simulink model "gm_hybrid_lht"  (R2019b)
settings: Solver=FixedStepDiscrete  StartTime=0.0  StopTime=inf  FixedStep=1/120e6  RelTol=1e-3
undefined symbols (not defined in the file or in its folder): bt, height, nTheta, width
libraries: hdlsllib x352, simulink x286, hdlmdlgenlib x7, dspsrcs4 x1
(part 2 of 12)

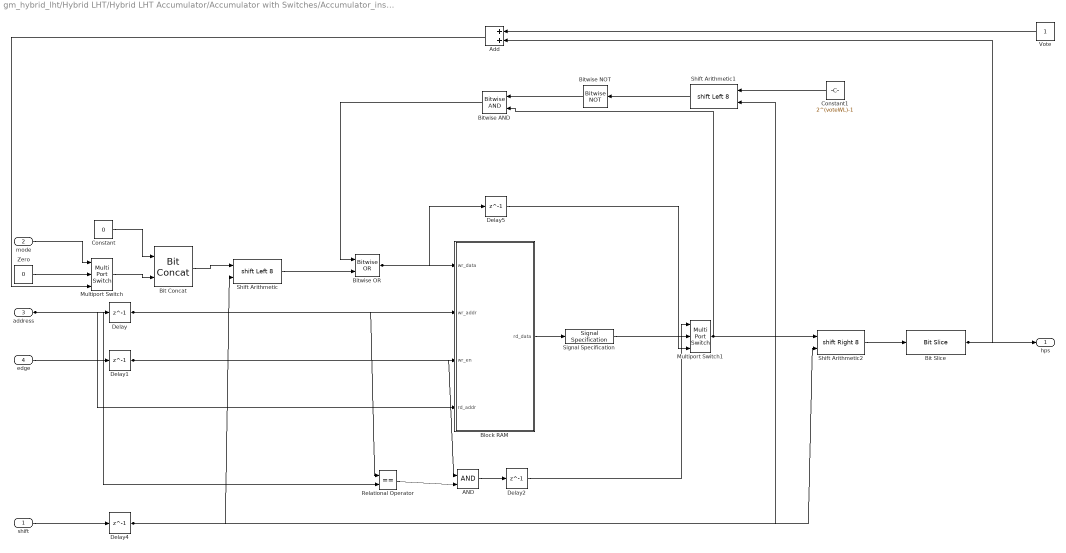
== system gm_hybrid_lht/Hybrid LHT/Hybrid LHT Accumulator/Accumulator with Switches/Accumulator_instance1 ==
  shift : Inport  OutDataTypeStr=fixdt(0, 6, 0)  PortDimensions=1  SampleTime=8.33333333333333e-09
  mode : Inport  Port=2  OutDataTypeStr=boolean  PortDimensions=1  SampleTime=8.33333333333333e-09
  address : Inport  Port=3  OutDataTypeStr=fixdt(0, 11, 0)  PortDimensions=1  SampleTime=8.33333333333333e-09
  edge : Inport  Port=4  OutDataTypeStr=boolean  PortDimensions=1  SampleTime=8.33333333333333e-09
  AND : Logic  IconShape=distinctive  AllPortsSameDT=off  OutDataTypeStr=boolean
  Add : Sum  OutDataTypeStr=fixdt(0, ceil(log2(maxRho*2)), 0)
  Bit Concat : hdlsllib/Logic and Bit Operations/Bit Concat  numInputs=2
      settings: SourceProductName=Simulink
  Bit Slice : hdlsllib/Logic and Bit Operations/Bit Slice  lidx=voteWL-1  ridx=0
  Bitwise AND : simulink/Logic and Bit Operations/Bitwise Operator  logicop=AND  UseBitMask=off  NumInputPorts=2  BitMask=bin2dec('11011001')  BitMaskRealWorld=Stored Integer
  Bitwise NOT : simulink/Logic and Bit Operations/Bitwise Operator  logicop=NOT  UseBitMask=off  BitMask=bin2dec('11011001')  BitMaskRealWorld=Stored Integer
  Bitwise OR : simulink/Logic and Bit Operations/Bitwise Operator  logicop=OR  UseBitMask=off  NumInputPorts=2  BitMask=bin2dec('11011001')  BitMaskRealWorld=Stored Integer
  Block RAM : Subsystem
  Constant : Constant  Value=0  OutDataTypeStr=fixdt(0, 36-voteWL, 0)  SampleTime=-1
  Constant1 : Constant  Value=2^(voteWL)-1  OutDataTypeStr=fixdt(0, 36, 0)  SampleTime=-1
  Delay{,1..2,4..5} (5 alike) : Delay  DelayLength=1
  Multiport Switch : MultiPortSwitch  DataPortOrder=Zero-based contiguous  Inputs=2  zeroidx=on
  Multiport Switch1 : MultiPortSwitch  DataPortOrder=Zero-based contiguous  Inputs=2  zeroidx=on
  Relational Operator : RelationalOperator  Operator===  OutDataTypeStr=boolean  RndMeth=Simplest
  Shift Arithmetic : ArithShift  BitShiftNumberSource=Input port  BitShiftNumber=8  BitShiftDirection=Left  DiagnosticForOORShift=Error
      settings: InputPortMap=u0,p1
  Shift Arithmetic1 : ArithShift  BitShiftNumberSource=Input port  BitShiftNumber=8  BitShiftDirection=Left  DiagnosticForOORShift=Error
      settings: InputPortMap=u0,p1
  Shift Arithmetic2 : ArithShift  BitShiftNumberSource=Input port  BitShiftNumber=8  BitShiftDirection=Right  DiagnosticForOORShift=Error
      settings: InputPortMap=u0,p1
  Signal Specification : SignalSpecification  OutDataTypeStr=fixdt(0, 36, 0)
  Vote : Constant  OutDataTypeStr=fixdt(0,1,0)  SampleTime=-1
  Zero : Constant  Value=0  OutDataTypeStr=fixdt(0,1,0)  SampleTime=-1
  hps : Outport
  wires:
  Zero/1 -> Multiport Switch/2
  Vote/1 -> Add/1
  Shift Arithmetic1/1 -> Bitwise NOT/1
  Relational Operator/1 -> AND/2
  Delay4/1 -> Shift Arithmetic1/2, Shift Arithmetic/2, Shift Arithmetic2/2
  Delay2/1 -> Multiport Switch1/1
  Delay1/1 -> AND/1, Block RAM/3(wr_en)
  Delay/1 -> Relational Operator/1, Block RAM/2(wr_addr)
  Constant1/1 -> Shift Arithmetic1/1
  Constant/1 -> Bit Concat/1
  Bitwise NOT/1 -> Bitwise AND/1
  Bit Slice/1 -> hps/1, Add/2
  AND/1 -> Delay2/1
  shift/1 -> Delay4/1
  mode/1 -> Multiport Switch/1
  address/1 -> Relational Operator/2, Delay/1, Block RAM/4(rd_addr)
  edge/1 -> Delay1/1
  Delay5/1 -> Multiport Switch1/3
  Shift Arithmetic/1 -> Bitwise OR/2
  Bit Concat/1 -> Shift Arithmetic/1
  Multiport Switch/1 -> Bit Concat/2
  Add/1 -> Multiport Switch/3
  Shift Arithmetic2/1 -> Bit Slice/1
  Bitwise AND/1 -> Bitwise OR/1
  Bitwise OR/1 -> Delay5/1, Block RAM/1(wr_data)
  Signal Specification/1 -> Multiport Switch1/2
  Multiport Switch1/1 -> Bitwise AND/2, Shift Arithmetic2/1
  Block RAM/1(rd_data) -> Signal Specification/1

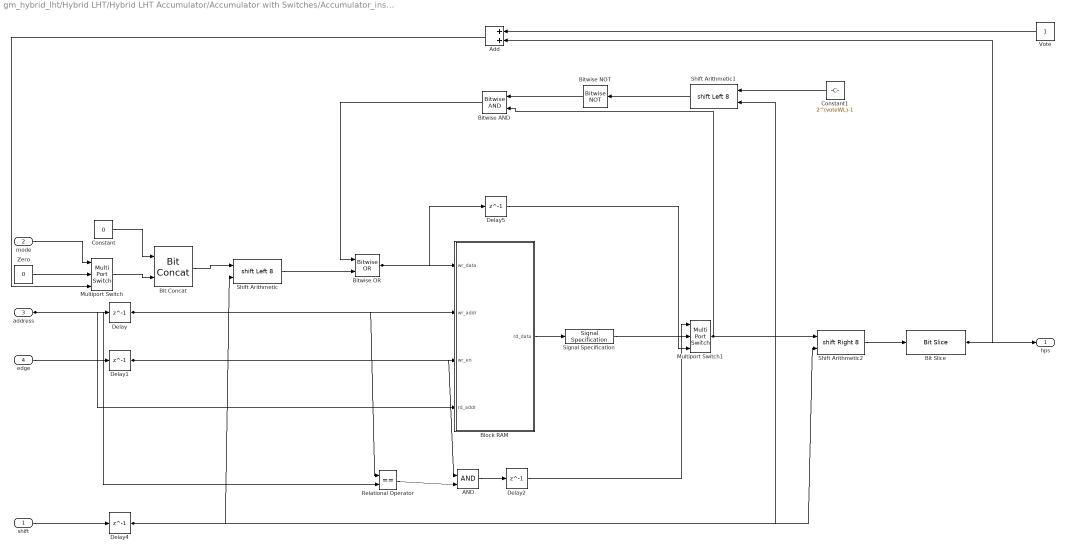
== system gm_hybrid_lht/Hybrid LHT/Hybrid LHT Accumulator/Accumulator with Switches/Accumulator_instance10 ==
  shift : Inport  OutDataTypeStr=fixdt(0, 6, 0)  PortDimensions=1  SampleTime=8.33333333333333e-09
  mode : Inport  Port=2  OutDataTypeStr=boolean  PortDimensions=1  SampleTime=8.33333333333333e-09
  address : Inport  Port=3  OutDataTypeStr=fixdt(0, 11, 0)  PortDimensions=1  SampleTime=8.33333333333333e-09
  edge : Inport  Port=4  OutDataTypeStr=boolean  PortDimensions=1  SampleTime=8.33333333333333e-09
  AND : Logic  IconShape=distinctive  AllPortsSameDT=off  OutDataTypeStr=boolean
  Add : Sum  OutDataTypeStr=fixdt(0, ceil(log2(maxRho*2)), 0)
  Bit Concat : hdlsllib/Logic and Bit Operations/Bit Concat  numInputs=2
      settings: SourceProductName=Simulink
  Bit Slice : hdlsllib/Logic and Bit Operations/Bit Slice  lidx=voteWL-1  ridx=0
  Bitwise AND : simulink/Logic and Bit Operations/Bitwise Operator  logicop=AND  UseBitMask=off  NumInputPorts=2  BitMask=bin2dec('11011001')  BitMaskRealWorld=Stored Integer
  Bitwise NOT : simulink/Logic and Bit Operations/Bitwise Operator  logicop=NOT  UseBitMask=off  BitMask=bin2dec('11011001')  BitMaskRealWorld=Stored Integer
  Bitwise OR : simulink/Logic and Bit Operations/Bitwise Operator  logicop=OR  UseBitMask=off  NumInputPorts=2  BitMask=bin2dec('11011001')  BitMaskRealWorld=Stored Integer
  Block RAM : Subsystem
  Constant : Constant  Value=0  OutDataTypeStr=fixdt(0, 36-voteWL, 0)  SampleTime=-1
  Constant1 : Constant  Value=2^(voteWL)-1  OutDataTypeStr=fixdt(0, 36, 0)  SampleTime=-1
  Delay{,1..2,4..5} (5 alike) : Delay  DelayLength=1
  Multiport Switch : MultiPortSwitch  DataPortOrder=Zero-based contiguous  Inputs=2  zeroidx=on
  Multiport Switch1 : MultiPortSwitch  DataPortOrder=Zero-based contiguous  Inputs=2  zeroidx=on
  Relational Operator : RelationalOperator  Operator===  OutDataTypeStr=boolean  RndMeth=Simplest
  Shift Arithmetic : ArithShift  BitShiftNumberSource=Input port  BitShiftNumber=8  BitShiftDirection=Left  DiagnosticForOORShift=Error
      settings: InputPortMap=u0,p1
  Shift Arithmetic1 : ArithShift  BitShiftNumberSource=Input port  BitShiftNumber=8  BitShiftDirection=Left  DiagnosticForOORShift=Error
      settings: InputPortMap=u0,p1
  Shift Arithmetic2 : ArithShift  BitShiftNumberSource=Input port  BitShiftNumber=8  BitShiftDirection=Right  DiagnosticForOORShift=Error
      settings: InputPortMap=u0,p1
  Signal Specification : SignalSpecification  OutDataTypeStr=fixdt(0, 36, 0)
  Vote : Constant  OutDataTypeStr=fixdt(0,1,0)  SampleTime=-1
  Zero : Constant  Value=0  OutDataTypeStr=fixdt(0,1,0)  SampleTime=-1
  hps : Outport
  wires:
  Block RAM/1(rd_data) -> Signal Specification/1
  Multiport Switch1/1 -> Shift Arithmetic2/1, Bitwise AND/2
  Signal Specification/1 -> Multiport Switch1/2
  Bitwise OR/1 -> Block RAM/1(wr_data), Delay5/1
  Bitwise AND/1 -> Bitwise OR/1
  Shift Arithmetic2/1 -> Bit Slice/1
  Add/1 -> Multiport Switch/3
  Multiport Switch/1 -> Bit Concat/2
  Bit Concat/1 -> Shift Arithmetic/1
  Shift Arithmetic/1 -> Bitwise OR/2
  Delay5/1 -> Multiport Switch1/3
  edge/1 -> Delay1/1
  address/1 -> Block RAM/4(rd_addr), Delay/1, Relational Operator/2
  mode/1 -> Multiport Switch/1
  shift/1 -> Delay4/1
  AND/1 -> Delay2/1
  Bit Slice/1 -> Add/2, hps/1
  Bitwise NOT/1 -> Bitwise AND/1
  Constant/1 -> Bit Concat/1
  Constant1/1 -> Shift Arithmetic1/1
  Delay/1 -> Block RAM/2(wr_addr), Relational Operator/1
  Delay1/1 -> Block RAM/3(wr_en), AND/1
  Delay2/1 -> Multiport Switch1/1
  Delay4/1 -> Shift Arithmetic2/2, Shift Arithmetic/2, Shift Arithmetic1/2
  Relational Operator/1 -> AND/2
  Shift Arithmetic1/1 -> Bitwise NOT/1
  Vote/1 -> Add/1
  Zero/1 -> Multiport Switch/2

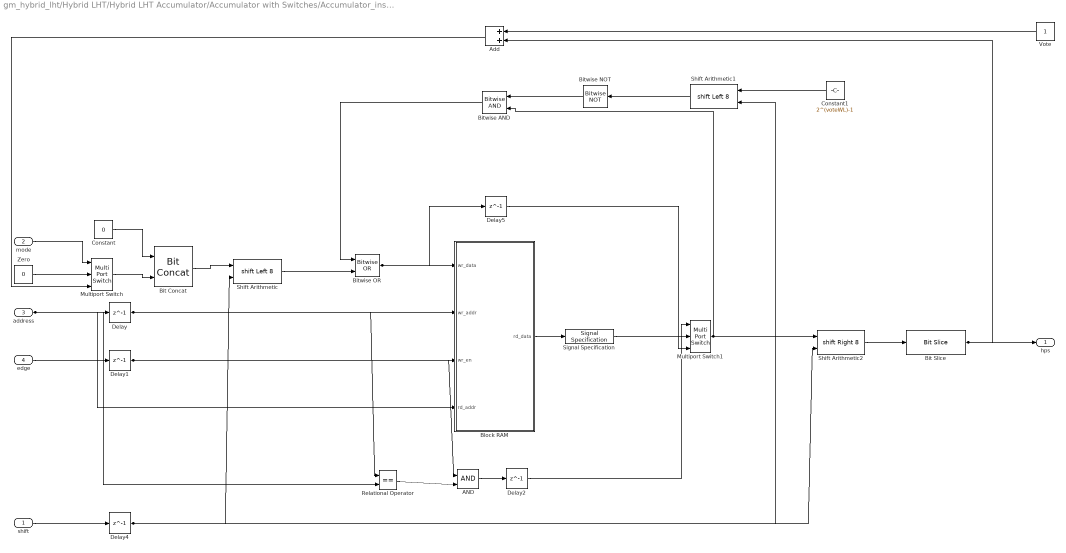
== system gm_hybrid_lht/Hybrid LHT/Hybrid LHT Accumulator/Accumulator with Switches/Accumulator_instance11 ==
  shift : Inport  OutDataTypeStr=fixdt(0, 6, 0)  PortDimensions=1  SampleTime=8.33333333333333e-09
  mode : Inport  Port=2  OutDataTypeStr=boolean  PortDimensions=1  SampleTime=8.33333333333333e-09
  address : Inport  Port=3  OutDataTypeStr=fixdt(0, 11, 0)  PortDimensions=1  SampleTime=8.33333333333333e-09
  edge : Inport  Port=4  OutDataTypeStr=boolean  PortDimensions=1  SampleTime=8.33333333333333e-09
  AND : Logic  IconShape=distinctive  AllPortsSameDT=off  OutDataTypeStr=boolean
  Add : Sum  OutDataTypeStr=fixdt(0, ceil(log2(maxRho*2)), 0)
  Bit Concat : hdlsllib/Logic and Bit Operations/Bit Concat  numInputs=2
      settings: SourceProductName=Simulink
  Bit Slice : hdlsllib/Logic and Bit Operations/Bit Slice  lidx=voteWL-1  ridx=0
  Bitwise AND : simulink/Logic and Bit Operations/Bitwise Operator  logicop=AND  UseBitMask=off  NumInputPorts=2  BitMask=bin2dec('11011001')  BitMaskRealWorld=Stored Integer
  Bitwise NOT : simulink/Logic and Bit Operations/Bitwise Operator  logicop=NOT  UseBitMask=off  BitMask=bin2dec('11011001')  BitMaskRealWorld=Stored Integer
  Bitwise OR : simulink/Logic and Bit Operations/Bitwise Operator  logicop=OR  UseBitMask=off  NumInputPorts=2  BitMask=bin2dec('11011001')  BitMaskRealWorld=Stored Integer
  Block RAM : Subsystem
  Constant : Constant  Value=0  OutDataTypeStr=fixdt(0, 36-voteWL, 0)  SampleTime=-1
  Constant1 : Constant  Value=2^(voteWL)-1  OutDataTypeStr=fixdt(0, 36, 0)  SampleTime=-1
  Delay{,1..2,4..5} (5 alike) : Delay  DelayLength=1
  Multiport Switch : MultiPortSwitch  DataPortOrder=Zero-based contiguous  Inputs=2  zeroidx=on
  Multiport Switch1 : MultiPortSwitch  DataPortOrder=Zero-based contiguous  Inputs=2  zeroidx=on
  Relational Operator : RelationalOperator  Operator===  OutDataTypeStr=boolean  RndMeth=Simplest
  Shift Arithmetic : ArithShift  BitShiftNumberSource=Input port  BitShiftNumber=8  BitShiftDirection=Left  DiagnosticForOORShift=Error
      settings: InputPortMap=u0,p1
  Shift Arithmetic1 : ArithShift  BitShiftNumberSource=Input port  BitShiftNumber=8  BitShiftDirection=Left  DiagnosticForOORShift=Error
      settings: InputPortMap=u0,p1
  Shift Arithmetic2 : ArithShift  BitShiftNumberSource=Input port  BitShiftNumber=8  BitShiftDirection=Right  DiagnosticForOORShift=Error
      settings: InputPortMap=u0,p1
  Signal Specification : SignalSpecification  OutDataTypeStr=fixdt(0, 36, 0)
  Vote : Constant  OutDataTypeStr=fixdt(0,1,0)  SampleTime=-1
  Zero : Constant  Value=0  OutDataTypeStr=fixdt(0,1,0)  SampleTime=-1
  hps : Outport
  wires:
  Block RAM/1(rd_data) -> Signal Specification/1
  Multiport Switch1/1 -> Shift Arithmetic2/1, Bitwise AND/2
  Signal Specification/1 -> Multiport Switch1/2
  Bitwise OR/1 -> Block RAM/1(wr_data), Delay5/1
  Bitwise AND/1 -> Bitwise OR/1
  Shift Arithmetic2/1 -> Bit Slice/1
  Add/1 -> Multiport Switch/3
  Multiport Switch/1 -> Bit Concat/2
  Bit Concat/1 -> Shift Arithmetic/1
  Shift Arithmetic/1 -> Bitwise OR/2
  Delay5/1 -> Multiport Switch1/3
  edge/1 -> Delay1/1
  address/1 -> Block RAM/4(rd_addr), Delay/1, Relational Operator/2
  mode/1 -> Multiport Switch/1
  shift/1 -> Delay4/1
  AND/1 -> Delay2/1
  Bit Slice/1 -> Add/2, hps/1
  Bitwise NOT/1 -> Bitwise AND/1
  Constant/1 -> Bit Concat/1
  Constant1/1 -> Shift Arithmetic1/1
  Delay/1 -> Block RAM/2(wr_addr), Relational Operator/1
  Delay1/1 -> Block RAM/3(wr_en), AND/1
  Delay2/1 -> Multiport Switch1/1
  Delay4/1 -> Shift Arithmetic2/2, Shift Arithmetic/2, Shift Arithmetic1/2
  Relational Operator/1 -> AND/2
  Shift Arithmetic1/1 -> Bitwise NOT/1
  Vote/1 -> Add/1
  Zero/1 -> Multiport Switch/2

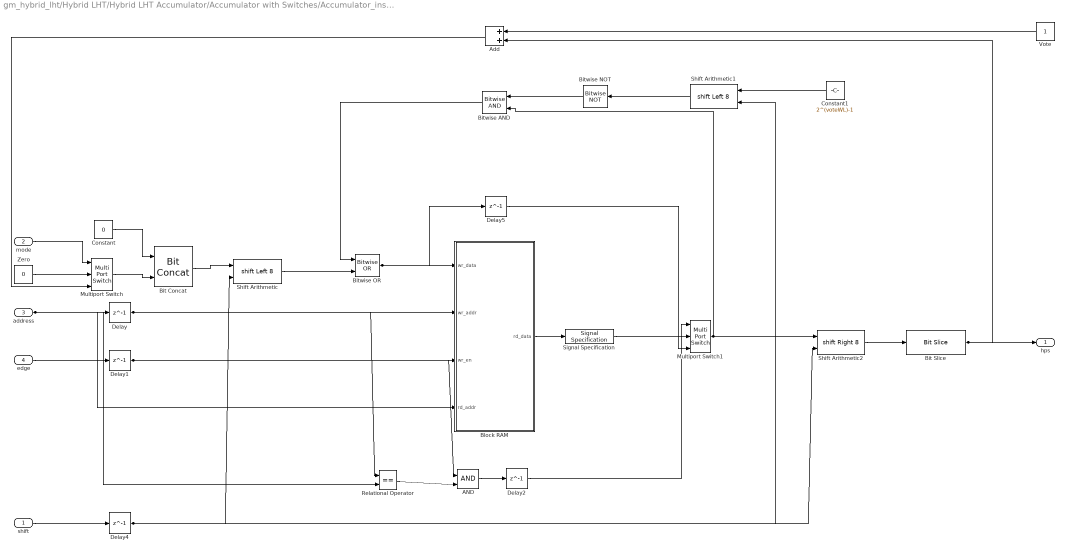
== system gm_hybrid_lht/Hybrid LHT/Hybrid LHT Accumulator/Accumulator with Switches/Accumulator_instance12 ==
  shift : Inport  OutDataTypeStr=fixdt(0, 6, 0)  PortDimensions=1  SampleTime=8.33333333333333e-09
  mode : Inport  Port=2  OutDataTypeStr=boolean  PortDimensions=1  SampleTime=8.33333333333333e-09
  address : Inport  Port=3  OutDataTypeStr=fixdt(0, 11, 0)  PortDimensions=1  SampleTime=8.33333333333333e-09
  edge : Inport  Port=4  OutDataTypeStr=boolean  PortDimensions=1  SampleTime=8.33333333333333e-09
  AND : Logic  IconShape=distinctive  AllPortsSameDT=off  OutDataTypeStr=boolean
  Add : Sum  OutDataTypeStr=fixdt(0, ceil(log2(maxRho*2)), 0)
  Bit Concat : hdlsllib/Logic and Bit Operations/Bit Concat  numInputs=2
      settings: SourceProductName=Simulink
  Bit Slice : hdlsllib/Logic and Bit Operations/Bit Slice  lidx=voteWL-1  ridx=0
  Bitwise AND : simulink/Logic and Bit Operations/Bitwise Operator  logicop=AND  UseBitMask=off  NumInputPorts=2  BitMask=bin2dec('11011001')  BitMaskRealWorld=Stored Integer
  Bitwise NOT : simulink/Logic and Bit Operations/Bitwise Operator  logicop=NOT  UseBitMask=off  BitMask=bin2dec('11011001')  BitMaskRealWorld=Stored Integer
  Bitwise OR : simulink/Logic and Bit Operations/Bitwise Operator  logicop=OR  UseBitMask=off  NumInputPorts=2  BitMask=bin2dec('11011001')  BitMaskRealWorld=Stored Integer
  Block RAM : Subsystem
  Constant : Constant  Value=0  OutDataTypeStr=fixdt(0, 36-voteWL, 0)  SampleTime=-1
  Constant1 : Constant  Value=2^(voteWL)-1  OutDataTypeStr=fixdt(0, 36, 0)  SampleTime=-1
  Delay{,1..2,4..5} (5 alike) : Delay  DelayLength=1
  Multiport Switch : MultiPortSwitch  DataPortOrder=Zero-based contiguous  Inputs=2  zeroidx=on
  Multiport Switch1 : MultiPortSwitch  DataPortOrder=Zero-based contiguous  Inputs=2  zeroidx=on
  Relational Operator : RelationalOperator  Operator===  OutDataTypeStr=boolean  RndMeth=Simplest
  Shift Arithmetic : ArithShift  BitShiftNumberSource=Input port  BitShiftNumber=8  BitShiftDirection=Left  DiagnosticForOORShift=Error
      settings: InputPortMap=u0,p1
  Shift Arithmetic1 : ArithShift  BitShiftNumberSource=Input port  BitShiftNumber=8  BitShiftDirection=Left  DiagnosticForOORShift=Error
      settings: InputPortMap=u0,p1
  Shift Arithmetic2 : ArithShift  BitShiftNumberSource=Input port  BitShiftNumber=8  BitShiftDirection=Right  DiagnosticForOORShift=Error
      settings: InputPortMap=u0,p1
  Signal Specification : SignalSpecification  OutDataTypeStr=fixdt(0, 36, 0)
  Vote : Constant  OutDataTypeStr=fixdt(0,1,0)  SampleTime=-1
  Zero : Constant  Value=0  OutDataTypeStr=fixdt(0,1,0)  SampleTime=-1
  hps : Outport
  wires:
  Block RAM/1(rd_data) -> Signal Specification/1
  Multiport Switch1/1 -> Shift Arithmetic2/1, Bitwise AND/2
  Signal Specification/1 -> Multiport Switch1/2
  Bitwise OR/1 -> Block RAM/1(wr_data), Delay5/1
  Bitwise AND/1 -> Bitwise OR/1
  Shift Arithmetic2/1 -> Bit Slice/1
  Add/1 -> Multiport Switch/3
  Multiport Switch/1 -> Bit Concat/2
  Bit Concat/1 -> Shift Arithmetic/1
  Shift Arithmetic/1 -> Bitwise OR/2
  Delay5/1 -> Multiport Switch1/3
  edge/1 -> Delay1/1
  address/1 -> Block RAM/4(rd_addr), Delay/1, Relational Operator/2
  mode/1 -> Multiport Switch/1
  shift/1 -> Delay4/1
  AND/1 -> Delay2/1
  Bit Slice/1 -> Add/2, hps/1
  Bitwise NOT/1 -> Bitwise AND/1
  Constant/1 -> Bit Concat/1
  Constant1/1 -> Shift Arithmetic1/1
  Delay/1 -> Block RAM/2(wr_addr), Relational Operator/1
  Delay1/1 -> Block RAM/3(wr_en), AND/1
  Delay2/1 -> Multiport Switch1/1
  Delay4/1 -> Shift Arithmetic2/2, Shift Arithmetic/2, Shift Arithmetic1/2
  Relational Operator/1 -> AND/2
  Shift Arithmetic1/1 -> Bitwise NOT/1
  Vote/1 -> Add/1
  Zero/1 -> Multiport Switch/2

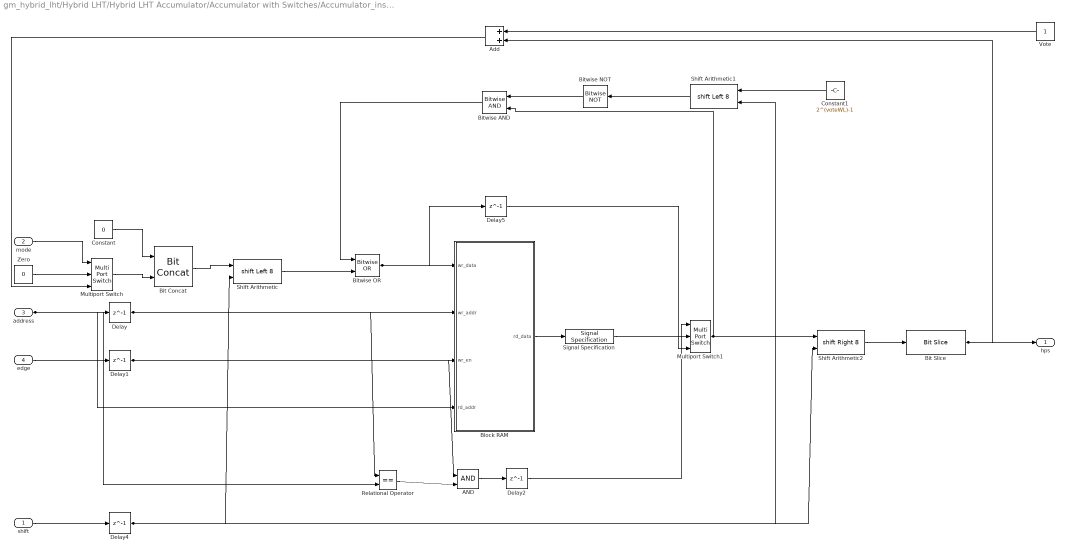
== system gm_hybrid_lht/Hybrid LHT/Hybrid LHT Accumulator/Accumulator with Switches/Accumulator_instance13 ==
  shift : Inport  OutDataTypeStr=fixdt(0, 6, 0)  PortDimensions=1  SampleTime=8.33333333333333e-09
  mode : Inport  Port=2  OutDataTypeStr=boolean  PortDimensions=1  SampleTime=8.33333333333333e-09
  address : Inport  Port=3  OutDataTypeStr=fixdt(0, 11, 0)  PortDimensions=1  SampleTime=8.33333333333333e-09
  edge : Inport  Port=4  OutDataTypeStr=boolean  PortDimensions=1  SampleTime=8.33333333333333e-09
  AND : Logic  IconShape=distinctive  AllPortsSameDT=off  OutDataTypeStr=boolean
  Add : Sum  OutDataTypeStr=fixdt(0, ceil(log2(maxRho*2)), 0)
  Bit Concat : hdlsllib/Logic and Bit Operations/Bit Concat  numInputs=2
      settings: SourceProductName=Simulink
  Bit Slice : hdlsllib/Logic and Bit Operations/Bit Slice  lidx=voteWL-1  ridx=0
  Bitwise AND : simulink/Logic and Bit Operations/Bitwise Operator  logicop=AND  UseBitMask=off  NumInputPorts=2  BitMask=bin2dec('11011001')  BitMaskRealWorld=Stored Integer
  Bitwise NOT : simulink/Logic and Bit Operations/Bitwise Operator  logicop=NOT  UseBitMask=off  BitMask=bin2dec('11011001')  BitMaskRealWorld=Stored Integer
  Bitwise OR : simulink/Logic and Bit Operations/Bitwise Operator  logicop=OR  UseBitMask=off  NumInputPorts=2  BitMask=bin2dec('11011001')  BitMaskRealWorld=Stored Integer
  Block RAM : Subsystem
  Constant : Constant  Value=0  OutDataTypeStr=fixdt(0, 36-voteWL, 0)  SampleTime=-1
  Constant1 : Constant  Value=2^(voteWL)-1  OutDataTypeStr=fixdt(0, 36, 0)  SampleTime=-1
  Delay{,1..2,4..5} (5 alike) : Delay  DelayLength=1
  Multiport Switch : MultiPortSwitch  DataPortOrder=Zero-based contiguous  Inputs=2  zeroidx=on
  Multiport Switch1 : MultiPortSwitch  DataPortOrder=Zero-based contiguous  Inputs=2  zeroidx=on
  Relational Operator : RelationalOperator  Operator===  OutDataTypeStr=boolean  RndMeth=Simplest
  Shift Arithmetic : ArithShift  BitShiftNumberSource=Input port  BitShiftNumber=8  BitShiftDirection=Left  DiagnosticForOORShift=Error
      settings: InputPortMap=u0,p1
  Shift Arithmetic1 : ArithShift  BitShiftNumberSource=Input port  BitShiftNumber=8  BitShiftDirection=Left  DiagnosticForOORShift=Error
      settings: InputPortMap=u0,p1
  Shift Arithmetic2 : ArithShift  BitShiftNumberSource=Input port  BitShiftNumber=8  BitShiftDirection=Right  DiagnosticForOORShift=Error
      settings: InputPortMap=u0,p1
  Signal Specification : SignalSpecification  OutDataTypeStr=fixdt(0, 36, 0)
  Vote : Constant  OutDataTypeStr=fixdt(0,1,0)  SampleTime=-1
  Zero : Constant  Value=0  OutDataTypeStr=fixdt(0,1,0)  SampleTime=-1
  hps : Outport
  wires:
  Block RAM/1(rd_data) -> Signal Specification/1
  Multiport Switch1/1 -> Shift Arithmetic2/1, Bitwise AND/2
  Signal Specification/1 -> Multiport Switch1/2
  Bitwise OR/1 -> Block RAM/1(wr_data), Delay5/1
  Bitwise AND/1 -> Bitwise OR/1
  Shift Arithmetic2/1 -> Bit Slice/1
  Add/1 -> Multiport Switch/3
  Multiport Switch/1 -> Bit Concat/2
  Bit Concat/1 -> Shift Arithmetic/1
  Shift Arithmetic/1 -> Bitwise OR/2
  Delay5/1 -> Multiport Switch1/3
  edge/1 -> Delay1/1
  address/1 -> Block RAM/4(rd_addr), Delay/1, Relational Operator/2
  mode/1 -> Multiport Switch/1
  shift/1 -> Delay4/1
  AND/1 -> Delay2/1
  Bit Slice/1 -> Add/2, hps/1
  Bitwise NOT/1 -> Bitwise AND/1
  Constant/1 -> Bit Concat/1
  Constant1/1 -> Shift Arithmetic1/1
  Delay/1 -> Block RAM/2(wr_addr), Relational Operator/1
  Delay1/1 -> Block RAM/3(wr_en), AND/1
  Delay2/1 -> Multiport Switch1/1
  Delay4/1 -> Shift Arithmetic2/2, Shift Arithmetic/2, Shift Arithmetic1/2
  Relational Operator/1 -> AND/2
  Shift Arithmetic1/1 -> Bitwise NOT/1
  Vote/1 -> Add/1
  Zero/1 -> Multiport Switch/2

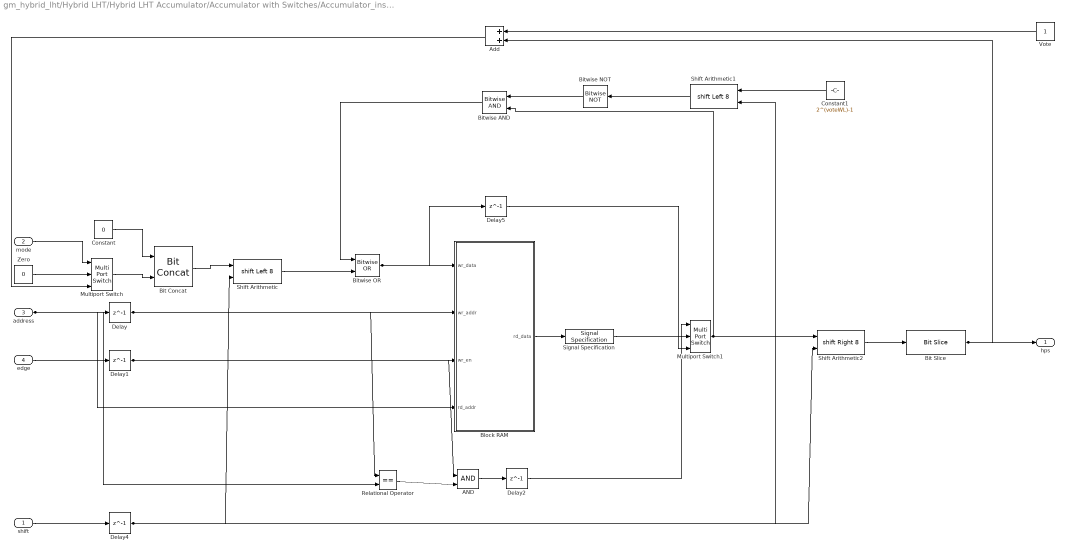
== system gm_hybrid_lht/Hybrid LHT/Hybrid LHT Accumulator/Accumulator with Switches/Accumulator_instance14 ==
  shift : Inport  OutDataTypeStr=fixdt(0, 6, 0)  PortDimensions=1  SampleTime=8.33333333333333e-09
  mode : Inport  Port=2  OutDataTypeStr=boolean  PortDimensions=1  SampleTime=8.33333333333333e-09
  address : Inport  Port=3  OutDataTypeStr=fixdt(0, 11, 0)  PortDimensions=1  SampleTime=8.33333333333333e-09
  edge : Inport  Port=4  OutDataTypeStr=boolean  PortDimensions=1  SampleTime=8.33333333333333e-09
  AND : Logic  IconShape=distinctive  AllPortsSameDT=off  OutDataTypeStr=boolean
  Add : Sum  OutDataTypeStr=fixdt(0, ceil(log2(maxRho*2)), 0)
  Bit Concat : hdlsllib/Logic and Bit Operations/Bit Concat  numInputs=2
      settings: SourceProductName=Simulink
  Bit Slice : hdlsllib/Logic and Bit Operations/Bit Slice  lidx=voteWL-1  ridx=0
  Bitwise AND : simulink/Logic and Bit Operations/Bitwise Operator  logicop=AND  UseBitMask=off  NumInputPorts=2  BitMask=bin2dec('11011001')  BitMaskRealWorld=Stored Integer
  Bitwise NOT : simulink/Logic and Bit Operations/Bitwise Operator  logicop=NOT  UseBitMask=off  BitMask=bin2dec('11011001')  BitMaskRealWorld=Stored Integer
  Bitwise OR : simulink/Logic and Bit Operations/Bitwise Operator  logicop=OR  UseBitMask=off  NumInputPorts=2  BitMask=bin2dec('11011001')  BitMaskRealWorld=Stored Integer
  Block RAM : Subsystem
  Constant : Constant  Value=0  OutDataTypeStr=fixdt(0, 36-voteWL, 0)  SampleTime=-1
  Constant1 : Constant  Value=2^(voteWL)-1  OutDataTypeStr=fixdt(0, 36, 0)  SampleTime=-1
  Delay{,1..2,4..5} (5 alike) : Delay  DelayLength=1
  Multiport Switch : MultiPortSwitch  DataPortOrder=Zero-based contiguous  Inputs=2  zeroidx=on
  Multiport Switch1 : MultiPortSwitch  DataPortOrder=Zero-based contiguous  Inputs=2  zeroidx=on
  Relational Operator : RelationalOperator  Operator===  OutDataTypeStr=boolean  RndMeth=Simplest
  Shift Arithmetic : ArithShift  BitShiftNumberSource=Input port  BitShiftNumber=8  BitShiftDirection=Left  DiagnosticForOORShift=Error
      settings: InputPortMap=u0,p1
  Shift Arithmetic1 : ArithShift  BitShiftNumberSource=Input port  BitShiftNumber=8  BitShiftDirection=Left  DiagnosticForOORShift=Error
      settings: InputPortMap=u0,p1
  Shift Arithmetic2 : ArithShift  BitShiftNumberSource=Input port  BitShiftNumber=8  BitShiftDirection=Right  DiagnosticForOORShift=Error
      settings: InputPortMap=u0,p1
  Signal Specification : SignalSpecification  OutDataTypeStr=fixdt(0, 36, 0)
  Vote : Constant  OutDataTypeStr=fixdt(0,1,0)  SampleTime=-1
  Zero : Constant  Value=0  OutDataTypeStr=fixdt(0,1,0)  SampleTime=-1
  hps : Outport
  wires:
  Block RAM/1(rd_data) -> Signal Specification/1
  Multiport Switch1/1 -> Shift Arithmetic2/1, Bitwise AND/2
  Signal Specification/1 -> Multiport Switch1/2
  Bitwise OR/1 -> Block RAM/1(wr_data), Delay5/1
  Bitwise AND/1 -> Bitwise OR/1
  Shift Arithmetic2/1 -> Bit Slice/1
  Add/1 -> Multiport Switch/3
  Multiport Switch/1 -> Bit Concat/2
  Bit Concat/1 -> Shift Arithmetic/1
  Shift Arithmetic/1 -> Bitwise OR/2
  Delay5/1 -> Multiport Switch1/3
  edge/1 -> Delay1/1
  address/1 -> Block RAM/4(rd_addr), Delay/1, Relational Operator/2
  mode/1 -> Multiport Switch/1
  shift/1 -> Delay4/1
  AND/1 -> Delay2/1
  Bit Slice/1 -> Add/2, hps/1
  Bitwise NOT/1 -> Bitwise AND/1
  Constant/1 -> Bit Concat/1
  Constant1/1 -> Shift Arithmetic1/1
  Delay/1 -> Block RAM/2(wr_addr), Relational Operator/1
  Delay1/1 -> Block RAM/3(wr_en), AND/1
  Delay2/1 -> Multiport Switch1/1
  Delay4/1 -> Shift Arithmetic2/2, Shift Arithmetic/2, Shift Arithmetic1/2
  Relational Operator/1 -> AND/2
  Shift Arithmetic1/1 -> Bitwise NOT/1
  Vote/1 -> Add/1
  Zero/1 -> Multiport Switch/2

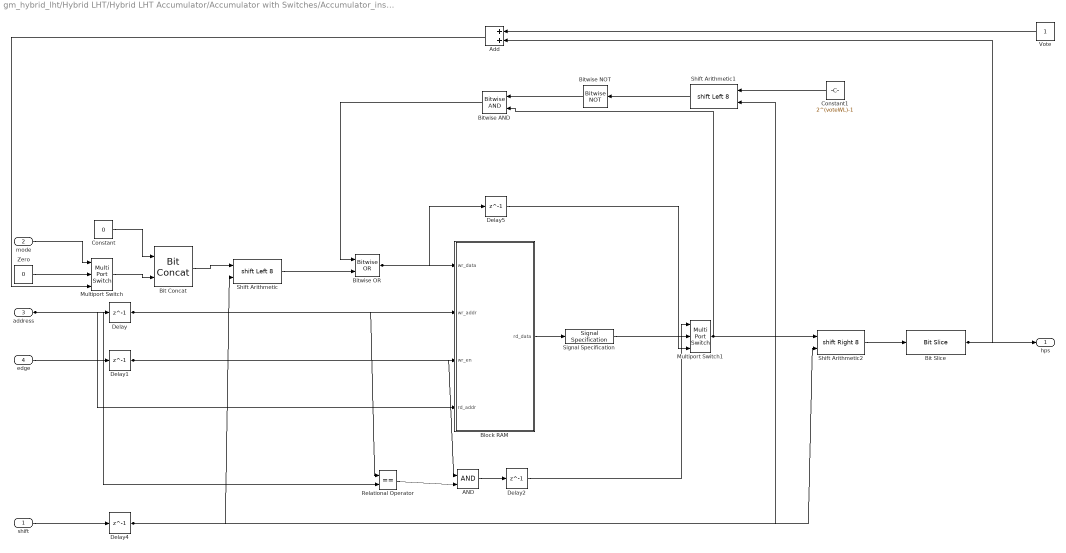
== system gm_hybrid_lht/Hybrid LHT/Hybrid LHT Accumulator/Accumulator with Switches/Accumulator_instance15 ==
  shift : Inport  OutDataTypeStr=fixdt(0, 6, 0)  PortDimensions=1  SampleTime=8.33333333333333e-09
  mode : Inport  Port=2  OutDataTypeStr=boolean  PortDimensions=1  SampleTime=8.33333333333333e-09
  address : Inport  Port=3  OutDataTypeStr=fixdt(0, 11, 0)  PortDimensions=1  SampleTime=8.33333333333333e-09
  edge : Inport  Port=4  OutDataTypeStr=boolean  PortDimensions=1  SampleTime=8.33333333333333e-09
  AND : Logic  IconShape=distinctive  AllPortsSameDT=off  OutDataTypeStr=boolean
  Add : Sum  OutDataTypeStr=fixdt(0, ceil(log2(maxRho*2)), 0)
  Bit Concat : hdlsllib/Logic and Bit Operations/Bit Concat  numInputs=2
      settings: SourceProductName=Simulink
  Bit Slice : hdlsllib/Logic and Bit Operations/Bit Slice  lidx=voteWL-1  ridx=0
  Bitwise AND : simulink/Logic and Bit Operations/Bitwise Operator  logicop=AND  UseBitMask=off  NumInputPorts=2  BitMask=bin2dec('11011001')  BitMaskRealWorld=Stored Integer
  Bitwise NOT : simulink/Logic and Bit Operations/Bitwise Operator  logicop=NOT  UseBitMask=off  BitMask=bin2dec('11011001')  BitMaskRealWorld=Stored Integer
  Bitwise OR : simulink/Logic and Bit Operations/Bitwise Operator  logicop=OR  UseBitMask=off  NumInputPorts=2  BitMask=bin2dec('11011001')  BitMaskRealWorld=Stored Integer
  Block RAM : Subsystem
  Constant : Constant  Value=0  OutDataTypeStr=fixdt(0, 36-voteWL, 0)  SampleTime=-1
  Constant1 : Constant  Value=2^(voteWL)-1  OutDataTypeStr=fixdt(0, 36, 0)  SampleTime=-1
  Delay{,1..2,4..5} (5 alike) : Delay  DelayLength=1
  Multiport Switch : MultiPortSwitch  DataPortOrder=Zero-based contiguous  Inputs=2  zeroidx=on
  Multiport Switch1 : MultiPortSwitch  DataPortOrder=Zero-based contiguous  Inputs=2  zeroidx=on
  Relational Operator : RelationalOperator  Operator===  OutDataTypeStr=boolean  RndMeth=Simplest
  Shift Arithmetic : ArithShift  BitShiftNumberSource=Input port  BitShiftNumber=8  BitShiftDirection=Left  DiagnosticForOORShift=Error
      settings: InputPortMap=u0,p1
  Shift Arithmetic1 : ArithShift  BitShiftNumberSource=Input port  BitShiftNumber=8  BitShiftDirection=Left  DiagnosticForOORShift=Error
      settings: InputPortMap=u0,p1
  Shift Arithmetic2 : ArithShift  BitShiftNumberSource=Input port  BitShiftNumber=8  BitShiftDirection=Right  DiagnosticForOORShift=Error
      settings: InputPortMap=u0,p1
  Signal Specification : SignalSpecification  OutDataTypeStr=fixdt(0, 36, 0)
  Vote : Constant  OutDataTypeStr=fixdt(0,1,0)  SampleTime=-1
  Zero : Constant  Value=0  OutDataTypeStr=fixdt(0,1,0)  SampleTime=-1
  hps : Outport
  wires:
  Block RAM/1(rd_data) -> Signal Specification/1
  Multiport Switch1/1 -> Shift Arithmetic2/1, Bitwise AND/2
  Signal Specification/1 -> Multiport Switch1/2
  Bitwise OR/1 -> Block RAM/1(wr_data), Delay5/1
  Bitwise AND/1 -> Bitwise OR/1
  Shift Arithmetic2/1 -> Bit Slice/1
  Add/1 -> Multiport Switch/3
  Multiport Switch/1 -> Bit Concat/2
  Bit Concat/1 -> Shift Arithmetic/1
  Shift Arithmetic/1 -> Bitwise OR/2
  Delay5/1 -> Multiport Switch1/3
  edge/1 -> Delay1/1
  address/1 -> Block RAM/4(rd_addr), Delay/1, Relational Operator/2
  mode/1 -> Multiport Switch/1
  shift/1 -> Delay4/1
  AND/1 -> Delay2/1
  Bit Slice/1 -> Add/2, hps/1
  Bitwise NOT/1 -> Bitwise AND/1
  Constant/1 -> Bit Concat/1
  Constant1/1 -> Shift Arithmetic1/1
  Delay/1 -> Block RAM/2(wr_addr), Relational Operator/1
  Delay1/1 -> Block RAM/3(wr_en), AND/1
  Delay2/1 -> Multiport Switch1/1
  Delay4/1 -> Shift Arithmetic2/2, Shift Arithmetic/2, Shift Arithmetic1/2
  Relational Operator/1 -> AND/2
  Shift Arithmetic1/1 -> Bitwise NOT/1
  Vote/1 -> Add/1
  Zero/1 -> Multiport Switch/2

== system gm_hybrid_lht/Hybrid LHT/Hybrid LHT Accumulator/Accumulator with Switches/Accumulator_instance16 ==
  shift : Inport  OutDataTypeStr=fixdt(0, 6, 0)  PortDimensions=1  SampleTime=8.33333333333333e-09
  mode : Inport  Port=2  OutDataTypeStr=boolean  PortDimensions=1  SampleTime=8.33333333333333e-09
  address : Inport  Port=3  OutDataTypeStr=fixdt(0, 11, 0)  PortDimensions=1  SampleTime=8.33333333333333e-09
  edge : Inport  Port=4  OutDataTypeStr=boolean  PortDimensions=1  SampleTime=8.33333333333333e-09
  AND : Logic  IconShape=distinctive  AllPortsSameDT=off  OutDataTypeStr=boolean
  Add : Sum  OutDataTypeStr=fixdt(0, ceil(log2(maxRho*2)), 0)
  Bit Concat : hdlsllib/Logic and Bit Operations/Bit Concat  numInputs=2
      settings: SourceProductName=Simulink
  Bit Slice : hdlsllib/Logic and Bit Operations/Bit Slice  lidx=voteWL-1  ridx=0
  Bitwise AND : simulink/Logic and Bit Operations/Bitwise Operator  logicop=AND  UseBitMask=off  NumInputPorts=2  BitMask=bin2dec('11011001')  BitMaskRealWorld=Stored Integer
  Bitwise NOT : simulink/Logic and Bit Operations/Bitwise Operator  logicop=NOT  UseBitMask=off  BitMask=bin2dec('11011001')  BitMaskRealWorld=Stored Integer
  Bitwise OR : simulink/Logic and Bit Operations/Bitwise Operator  logicop=OR  UseBitMask=off  NumInputPorts=2  BitMask=bin2dec('11011001')  BitMaskRealWorld=Stored Integer
  Block RAM : Subsystem
  Constant : Constant  Value=0  OutDataTypeStr=fixdt(0, 36-voteWL, 0)  SampleTime=-1
  Constant1 : Constant  Value=2^(voteWL)-1  OutDataTypeStr=fixdt(0, 36, 0)  SampleTime=-1
  Delay{,1..2,4..5} (5 alike) : Delay  DelayLength=1
  Multiport Switch : MultiPortSwitch  DataPortOrder=Zero-based contiguous  Inputs=2  zeroidx=on
  Multiport Switch1 : MultiPortSwitch  DataPortOrder=Zero-based contiguous  Inputs=2  zeroidx=on
  Relational Operator : RelationalOperator  Operator===  OutDataTypeStr=boolean  RndMeth=Simplest
  Shift Arithmetic : ArithShift  BitShiftNumberSource=Input port  BitShiftNumber=8  BitShiftDirection=Left  DiagnosticForOORShift=Error
      settings: InputPortMap=u0,p1
  Shift Arithmetic1 : ArithShift  BitShiftNumberSource=Input port  BitShiftNumber=8  BitShiftDirection=Left  DiagnosticForOORShift=Error
      settings: InputPortMap=u0,p1
  Shift Arithmetic2 : ArithShift  BitShiftNumberSource=Input port  BitShiftNumber=8  BitShiftDirection=Right  DiagnosticForOORShift=Error
      settings: InputPortMap=u0,p1
  Signal Specification : SignalSpecification  OutDataTypeStr=fixdt(0, 36, 0)
  Vote : Constant  OutDataTypeStr=fixdt(0,1,0)  SampleTime=-1
  Zero : Constant  Value=0  OutDataTypeStr=fixdt(0,1,0)  SampleTime=-1
  hps : Outport
  wires:
  Block RAM/1(rd_data) -> Signal Specification/1
  Multiport Switch1/1 -> Shift Arithmetic2/1, Bitwise AND/2
  Signal Specification/1 -> Multiport Switch1/2
  Bitwise OR/1 -> Block RAM/1(wr_data), Delay5/1
  Bitwise AND/1 -> Bitwise OR/1
  Shift Arithmetic2/1 -> Bit Slice/1
  Add/1 -> Multiport Switch/3
  Multiport Switch/1 -> Bit Concat/2
  Bit Concat/1 -> Shift Arithmetic/1
  Shift Arithmetic/1 -> Bitwise OR/2
  Delay5/1 -> Multiport Switch1/3
  edge/1 -> Delay1/1
  address/1 -> Block RAM/4(rd_addr), Delay/1, Relational Operator/2
  mode/1 -> Multiport Switch/1
  shift/1 -> Delay4/1
  AND/1 -> Delay2/1
  Bit Slice/1 -> Add/2, hps/1
  Bitwise NOT/1 -> Bitwise AND/1
  Constant/1 -> Bit Concat/1
  Constant1/1 -> Shift Arithmetic1/1
  Delay/1 -> Block RAM/2(wr_addr), Relational Operator/1
  Delay1/1 -> Block RAM/3(wr_en), AND/1
  Delay2/1 -> Multiport Switch1/1
  Delay4/1 -> Shift Arithmetic2/2, Shift Arithmetic/2, Shift Arithmetic1/2
  Relational Operator/1 -> AND/2
  Shift Arithmetic1/1 -> Bitwise NOT/1
  Vote/1 -> Add/1
  Zero/1 -> Multiport Switch/2

== system gm_hybrid_lht/Hybrid LHT/Hybrid LHT Accumulator/Accumulator with Switches/Accumulator_instance17 ==
  shift : Inport  OutDataTypeStr=fixdt(0, 6, 0)  PortDimensions=1  SampleTime=8.33333333333333e-09
  mode : Inport  Port=2  OutDataTypeStr=boolean  PortDimensions=1  SampleTime=8.33333333333333e-09
  address : Inport  Port=3  OutDataTypeStr=fixdt(0, 11, 0)  PortDimensions=1  SampleTime=8.33333333333333e-09
  edge : Inport  Port=4  OutDataTypeStr=boolean  PortDimensions=1  SampleTime=8.33333333333333e-09
  AND : Logic  IconShape=distinctive  AllPortsSameDT=off  OutDataTypeStr=boolean
  Add : Sum  OutDataTypeStr=fixdt(0, ceil(log2(maxRho*2)), 0)
  Bit Concat : hdlsllib/Logic and Bit Operations/Bit Concat  numInputs=2
      settings: SourceProductName=Simulink
  Bit Slice : hdlsllib/Logic and Bit Operations/Bit Slice  lidx=voteWL-1  ridx=0
  Bitwise AND : simulink/Logic and Bit Operations/Bitwise Operator  logicop=AND  UseBitMask=off  NumInputPorts=2  BitMask=bin2dec('11011001')  BitMaskRealWorld=Stored Integer
  Bitwise NOT : simulink/Logic and Bit Operations/Bitwise Operator  logicop=NOT  UseBitMask=off  BitMask=bin2dec('11011001')  BitMaskRealWorld=Stored Integer
  Bitwise OR : simulink/Logic and Bit Operations/Bitwise Operator  logicop=OR  UseBitMask=off  NumInputPorts=2  BitMask=bin2dec('11011001')  BitMaskRealWorld=Stored Integer
  Block RAM : Subsystem
  Constant : Constant  Value=0  OutDataTypeStr=fixdt(0, 36-voteWL, 0)  SampleTime=-1
  Constant1 : Constant  Value=2^(voteWL)-1  OutDataTypeStr=fixdt(0, 36, 0)  SampleTime=-1
  Delay{,1..2,4..5} (5 alike) : Delay  DelayLength=1
  Multiport Switch : MultiPortSwitch  DataPortOrder=Zero-based contiguous  Inputs=2  zeroidx=on
  Multiport Switch1 : MultiPortSwitch  DataPortOrder=Zero-based contiguous  Inputs=2  zeroidx=on
  Relational Operator : RelationalOperator  Operator===  OutDataTypeStr=boolean  RndMeth=Simplest
  Shift Arithmetic : ArithShift  BitShiftNumberSource=Input port  BitShiftNumber=8  BitShiftDirection=Left  DiagnosticForOORShift=Error
      settings: InputPortMap=u0,p1
  Shift Arithmetic1 : ArithShift  BitShiftNumberSource=Input port  BitShiftNumber=8  BitShiftDirection=Left  DiagnosticForOORShift=Error
      settings: InputPortMap=u0,p1
  Shift Arithmetic2 : ArithShift  BitShiftNumberSource=Input port  BitShiftNumber=8  BitShiftDirection=Right  DiagnosticForOORShift=Error
      settings: InputPortMap=u0,p1
  Signal Specification : SignalSpecification  OutDataTypeStr=fixdt(0, 36, 0)
  Vote : Constant  OutDataTypeStr=fixdt(0,1,0)  SampleTime=-1
  Zero : Constant  Value=0  OutDataTypeStr=fixdt(0,1,0)  SampleTime=-1
  hps : Outport
  wires:
  Block RAM/1(rd_data) -> Signal Specification/1
  Multiport Switch1/1 -> Shift Arithmetic2/1, Bitwise AND/2
  Signal Specification/1 -> Multiport Switch1/2
  Bitwise OR/1 -> Block RAM/1(wr_data), Delay5/1
  Bitwise AND/1 -> Bitwise OR/1
  Shift Arithmetic2/1 -> Bit Slice/1
  Add/1 -> Multiport Switch/3
  Multiport Switch/1 -> Bit Concat/2
  Bit Concat/1 -> Shift Arithmetic/1
  Shift Arithmetic/1 -> Bitwise OR/2
  Delay5/1 -> Multiport Switch1/3
  edge/1 -> Delay1/1
  address/1 -> Block RAM/4(rd_addr), Delay/1, Relational Operator/2
  mode/1 -> Multiport Switch/1
  shift/1 -> Delay4/1
  AND/1 -> Delay2/1
  Bit Slice/1 -> Add/2, hps/1
  Bitwise NOT/1 -> Bitwise AND/1
  Constant/1 -> Bit Concat/1
  Constant1/1 -> Shift Arithmetic1/1
  Delay/1 -> Block RAM/2(wr_addr), Relational Operator/1
  Delay1/1 -> Block RAM/3(wr_en), AND/1
  Delay2/1 -> Multiport Switch1/1
  Delay4/1 -> Shift Arithmetic2/2, Shift Arithmetic/2, Shift Arithmetic1/2
  Relational Operator/1 -> AND/2
  Shift Arithmetic1/1 -> Bitwise NOT/1
  Vote/1 -> Add/1
  Zero/1 -> Multiport Switch/2

== system gm_hybrid_lht/Hybrid LHT/Hybrid LHT Accumulator/Accumulator with Switches/Accumulator_instance18 ==
  shift : Inport  OutDataTypeStr=fixdt(0, 6, 0)  PortDimensions=1  SampleTime=8.33333333333333e-09
  mode : Inport  Port=2  OutDataTypeStr=boolean  PortDimensions=1  SampleTime=8.33333333333333e-09
  address : Inport  Port=3  OutDataTypeStr=fixdt(0, 11, 0)  PortDimensions=1  SampleTime=8.33333333333333e-09
  edge : Inport  Port=4  OutDataTypeStr=boolean  PortDimensions=1  SampleTime=8.33333333333333e-09
  AND : Logic  IconShape=distinctive  AllPortsSameDT=off  OutDataTypeStr=boolean
  Add : Sum  OutDataTypeStr=fixdt(0, ceil(log2(maxRho*2)), 0)
  Bit Concat : hdlsllib/Logic and Bit Operations/Bit Concat  numInputs=2
      settings: SourceProductName=Simulink
  Bit Slice : hdlsllib/Logic and Bit Operations/Bit Slice  lidx=voteWL-1  ridx=0
  Bitwise AND : simulink/Logic and Bit Operations/Bitwise Operator  logicop=AND  UseBitMask=off  NumInputPorts=2  BitMask=bin2dec('11011001')  BitMaskRealWorld=Stored Integer
  Bitwise NOT : simulink/Logic and Bit Operations/Bitwise Operator  logicop=NOT  UseBitMask=off  BitMask=bin2dec('11011001')  BitMaskRealWorld=Stored Integer
  Bitwise OR : simulink/Logic and Bit Operations/Bitwise Operator  logicop=OR  UseBitMask=off  NumInputPorts=2  BitMask=bin2dec('11011001')  BitMaskRealWorld=Stored Integer
  Block RAM : Subsystem
  Constant : Constant  Value=0  OutDataTypeStr=fixdt(0, 36-voteWL, 0)  SampleTime=-1
  Constant1 : Constant  Value=2^(voteWL)-1  OutDataTypeStr=fixdt(0, 36, 0)  SampleTime=-1
  Delay{,1..2,4..5} (5 alike) : Delay  DelayLength=1
  Multiport Switch : MultiPortSwitch  DataPortOrder=Zero-based contiguous  Inputs=2  zeroidx=on
  Multiport Switch1 : MultiPortSwitch  DataPortOrder=Zero-based contiguous  Inputs=2  zeroidx=on
  Relational Operator : RelationalOperator  Operator===  OutDataTypeStr=boolean  RndMeth=Simplest
  Shift Arithmetic : ArithShift  BitShiftNumberSource=Input port  BitShiftNumber=8  BitShiftDirection=Left  DiagnosticForOORShift=Error
      settings: InputPortMap=u0,p1
  Shift Arithmetic1 : ArithShift  BitShiftNumberSource=Input port  BitShiftNumber=8  BitShiftDirection=Left  DiagnosticForOORShift=Error
      settings: InputPortMap=u0,p1
  Shift Arithmetic2 : ArithShift  BitShiftNumberSource=Input port  BitShiftNumber=8  BitShiftDirection=Right  DiagnosticForOORShift=Error
      settings: InputPortMap=u0,p1
  Signal Specification : SignalSpecification  OutDataTypeStr=fixdt(0, 36, 0)
  Vote : Constant  OutDataTypeStr=fixdt(0,1,0)  SampleTime=-1
  Zero : Constant  Value=0  OutDataTypeStr=fixdt(0,1,0)  SampleTime=-1
  hps : Outport
  wires:
  Block RAM/1(rd_data) -> Signal Specification/1
  Multiport Switch1/1 -> Shift Arithmetic2/1, Bitwise AND/2
  Signal Specification/1 -> Multiport Switch1/2
  Bitwise OR/1 -> Block RAM/1(wr_data), Delay5/1
  Bitwise AND/1 -> Bitwise OR/1
  Shift Arithmetic2/1 -> Bit Slice/1
  Add/1 -> Multiport Switch/3
  Multiport Switch/1 -> Bit Concat/2
  Bit Concat/1 -> Shift Arithmetic/1
  Shift Arithmetic/1 -> Bitwise OR/2
  Delay5/1 -> Multiport Switch1/3
  edge/1 -> Delay1/1
  address/1 -> Block RAM/4(rd_addr), Delay/1, Relational Operator/2
  mode/1 -> Multiport Switch/1
  shift/1 -> Delay4/1
  AND/1 -> Delay2/1
  Bit Slice/1 -> Add/2, hps/1
  Bitwise NOT/1 -> Bitwise AND/1
  Constant/1 -> Bit Concat/1
  Constant1/1 -> Shift Arithmetic1/1
  Delay/1 -> Block RAM/2(wr_addr), Relational Operator/1
  Delay1/1 -> Block RAM/3(wr_en), AND/1
  Delay2/1 -> Multiport Switch1/1
  Delay4/1 -> Shift Arithmetic2/2, Shift Arithmetic/2, Shift Arithmetic1/2
  Relational Operator/1 -> AND/2
  Shift Arithmetic1/1 -> Bitwise NOT/1
  Vote/1 -> Add/1
  Zero/1 -> Multiport Switch/2

== system gm_hybrid_lht/Hybrid LHT/Hybrid LHT Accumulator/Accumulator with Switches/Accumulator_instance19 ==
  shift : Inport  OutDataTypeStr=fixdt(0, 6, 0)  PortDimensions=1  SampleTime=8.33333333333333e-09
  mode : Inport  Port=2  OutDataTypeStr=boolean  PortDimensions=1  SampleTime=8.33333333333333e-09
  address : Inport  Port=3  OutDataTypeStr=fixdt(0, 11, 0)  PortDimensions=1  SampleTime=8.33333333333333e-09
  edge : Inport  Port=4  OutDataTypeStr=boolean  PortDimensions=1  SampleTime=8.33333333333333e-09
  AND : Logic  IconShape=distinctive  AllPortsSameDT=off  OutDataTypeStr=boolean
  Add : Sum  OutDataTypeStr=fixdt(0, ceil(log2(maxRho*2)), 0)
  Bit Concat : hdlsllib/Logic and Bit Operations/Bit Concat  numInputs=2
      settings: SourceProductName=Simulink
  Bit Slice : hdlsllib/Logic and Bit Operations/Bit Slice  lidx=voteWL-1  ridx=0
  Bitwise AND : simulink/Logic and Bit Operations/Bitwise Operator  logicop=AND  UseBitMask=off  NumInputPorts=2  BitMask=bin2dec('11011001')  BitMaskRealWorld=Stored Integer
  Bitwise NOT : simulink/Logic and Bit Operations/Bitwise Operator  logicop=NOT  UseBitMask=off  BitMask=bin2dec('11011001')  BitMaskRealWorld=Stored Integer
  Bitwise OR : simulink/Logic and Bit Operations/Bitwise Operator  logicop=OR  UseBitMask=off  NumInputPorts=2  BitMask=bin2dec('11011001')  BitMaskRealWorld=Stored Integer
  Block RAM : Subsystem
  Constant : Constant  Value=0  OutDataTypeStr=fixdt(0, 36-voteWL, 0)  SampleTime=-1
  Constant1 : Constant  Value=2^(voteWL)-1  OutDataTypeStr=fixdt(0, 36, 0)  SampleTime=-1
  Delay{,1..2,4..5} (5 alike) : Delay  DelayLength=1
  Multiport Switch : MultiPortSwitch  DataPortOrder=Zero-based contiguous  Inputs=2  zeroidx=on
  Multiport Switch1 : MultiPortSwitch  DataPortOrder=Zero-based contiguous  Inputs=2  zeroidx=on
  Relational Operator : RelationalOperator  Operator===  OutDataTypeStr=boolean  RndMeth=Simplest
  Shift Arithmetic : ArithShift  BitShiftNumberSource=Input port  BitShiftNumber=8  BitShiftDirection=Left  DiagnosticForOORShift=Error
      settings: InputPortMap=u0,p1
  Shift Arithmetic1 : ArithShift  BitShiftNumberSource=Input port  BitShiftNumber=8  BitShiftDirection=Left  DiagnosticForOORShift=Error
      settings: InputPortMap=u0,p1
  Shift Arithmetic2 : ArithShift  BitShiftNumberSource=Input port  BitShiftNumber=8  BitShiftDirection=Right  DiagnosticForOORShift=Error
      settings: InputPortMap=u0,p1
  Signal Specification : SignalSpecification  OutDataTypeStr=fixdt(0, 36, 0)
  Vote : Constant  OutDataTypeStr=fixdt(0,1,0)  SampleTime=-1
  Zero : Constant  Value=0  OutDataTypeStr=fixdt(0,1,0)  SampleTime=-1
  hps : Outport
  wires:
  Block RAM/1(rd_data) -> Signal Specification/1
  Multiport Switch1/1 -> Shift Arithmetic2/1, Bitwise AND/2
  Signal Specification/1 -> Multiport Switch1/2
  Bitwise OR/1 -> Block RAM/1(wr_data), Delay5/1
  Bitwise AND/1 -> Bitwise OR/1
  Shift Arithmetic2/1 -> Bit Slice/1
  Add/1 -> Multiport Switch/3
  Multiport Switch/1 -> Bit Concat/2
  Bit Concat/1 -> Shift Arithmetic/1
  Shift Arithmetic/1 -> Bitwise OR/2
  Delay5/1 -> Multiport Switch1/3
  edge/1 -> Delay1/1
  address/1 -> Block RAM/4(rd_addr), Delay/1, Relational Operator/2
  mode/1 -> Multiport Switch/1
  shift/1 -> Delay4/1
  AND/1 -> Delay2/1
  Bit Slice/1 -> Add/2, hps/1
  Bitwise NOT/1 -> Bitwise AND/1
  Constant/1 -> Bit Concat/1
  Constant1/1 -> Shift Arithmetic1/1
  Delay/1 -> Block RAM/2(wr_addr), Relational Operator/1
  Delay1/1 -> Block RAM/3(wr_en), AND/1
  Delay2/1 -> Multiport Switch1/1
  Delay4/1 -> Shift Arithmetic2/2, Shift Arithmetic/2, Shift Arithmetic1/2
  Relational Operator/1 -> AND/2
  Shift Arithmetic1/1 -> Bitwise NOT/1
  Vote/1 -> Add/1
  Zero/1 -> Multiport Switch/2

== system gm_hybrid_lht/Hybrid LHT/Hybrid LHT Accumulator/Accumulator with Switches/Accumulator_instance2 ==
  shift : Inport  OutDataTypeStr=fixdt(0, 6, 0)  PortDimensions=1  SampleTime=8.33333333333333e-09
  mode : Inport  Port=2  OutDataTypeStr=boolean  PortDimensions=1  SampleTime=8.33333333333333e-09
  address : Inport  Port=3  OutDataTypeStr=fixdt(0, 11, 0)  PortDimensions=1  SampleTime=8.33333333333333e-09
  edge : Inport  Port=4  OutDataTypeStr=boolean  PortDimensions=1  SampleTime=8.33333333333333e-09
  AND : Logic  IconShape=distinctive  AllPortsSameDT=off  OutDataTypeStr=boolean
  Add : Sum  OutDataTypeStr=fixdt(0, ceil(log2(maxRho*2)), 0)
  Bit Concat : hdlsllib/Logic and Bit Operations/Bit Concat  numInputs=2
      settings: SourceProductName=Simulink
  Bit Slice : hdlsllib/Logic and Bit Operations/Bit Slice  lidx=voteWL-1  ridx=0
  Bitwise AND : simulink/Logic and Bit Operations/Bitwise Operator  logicop=AND  UseBitMask=off  NumInputPorts=2  BitMask=bin2dec('11011001')  BitMaskRealWorld=Stored Integer
  Bitwise NOT : simulink/Logic and Bit Operations/Bitwise Operator  logicop=NOT  UseBitMask=off  BitMask=bin2dec('11011001')  BitMaskRealWorld=Stored Integer
  Bitwise OR : simulink/Logic and Bit Operations/Bitwise Operator  logicop=OR  UseBitMask=off  NumInputPorts=2  BitMask=bin2dec('11011001')  BitMaskRealWorld=Stored Integer
  Block RAM : Subsystem
  Constant : Constant  Value=0  OutDataTypeStr=fixdt(0, 36-voteWL, 0)  SampleTime=-1
  Constant1 : Constant  Value=2^(voteWL)-1  OutDataTypeStr=fixdt(0, 36, 0)  SampleTime=-1
  Delay{,1..2,4..5} (5 alike) : Delay  DelayLength=1
  Multiport Switch : MultiPortSwitch  DataPortOrder=Zero-based contiguous  Inputs=2  zeroidx=on
  Multiport Switch1 : MultiPortSwitch  DataPortOrder=Zero-based contiguous  Inputs=2  zeroidx=on
  Relational Operator : RelationalOperator  Operator===  OutDataTypeStr=boolean  RndMeth=Simplest
  Shift Arithmetic : ArithShift  BitShiftNumberSource=Input port  BitShiftNumber=8  BitShiftDirection=Left  DiagnosticForOORShift=Error
      settings: InputPortMap=u0,p1
  Shift Arithmetic1 : ArithShift  BitShiftNumberSource=Input port  BitShiftNumber=8  BitShiftDirection=Left  DiagnosticForOORShift=Error
      settings: InputPortMap=u0,p1
  Shift Arithmetic2 : ArithShift  BitShiftNumberSource=Input port  BitShiftNumber=8  BitShiftDirection=Right  DiagnosticForOORShift=Error
      settings: InputPortMap=u0,p1
  Signal Specification : SignalSpecification  OutDataTypeStr=fixdt(0, 36, 0)
  Vote : Constant  OutDataTypeStr=fixdt(0,1,0)  SampleTime=-1
  Zero : Constant  Value=0  OutDataTypeStr=fixdt(0,1,0)  SampleTime=-1
  hps : Outport
  wires:
  Block RAM/1(rd_data) -> Signal Specification/1
  Multiport Switch1/1 -> Shift Arithmetic2/1, Bitwise AND/2
  Signal Specification/1 -> Multiport Switch1/2
  Bitwise OR/1 -> Block RAM/1(wr_data), Delay5/1
  Bitwise AND/1 -> Bitwise OR/1
  Shift Arithmetic2/1 -> Bit Slice/1
  Add/1 -> Multiport Switch/3
  Multiport Switch/1 -> Bit Concat/2
  Bit Concat/1 -> Shift Arithmetic/1
  Shift Arithmetic/1 -> Bitwise OR/2
  Delay5/1 -> Multiport Switch1/3
  edge/1 -> Delay1/1
  address/1 -> Block RAM/4(rd_addr), Delay/1, Relational Operator/2
  mode/1 -> Multiport Switch/1
  shift/1 -> Delay4/1
  AND/1 -> Delay2/1
  Bit Slice/1 -> Add/2, hps/1
  Bitwise NOT/1 -> Bitwise AND/1
  Constant/1 -> Bit Concat/1
  Constant1/1 -> Shift Arithmetic1/1
  Delay/1 -> Block RAM/2(wr_addr), Relational Operator/1
  Delay1/1 -> Block RAM/3(wr_en), AND/1
  Delay2/1 -> Multiport Switch1/1
  Delay4/1 -> Shift Arithmetic2/2, Shift Arithmetic/2, Shift Arithmetic1/2
  Relational Operator/1 -> AND/2
  Shift Arithmetic1/1 -> Bitwise NOT/1
  Vote/1 -> Add/1
  Zero/1 -> Multiport Switch/2

== system gm_hybrid_lht/Hybrid LHT/Hybrid LHT Accumulator/Accumulator with Switches/Accumulator_instance20 ==
  shift : Inport  OutDataTypeStr=fixdt(0, 6, 0)  PortDimensions=1  SampleTime=8.33333333333333e-09
  mode : Inport  Port=2  OutDataTypeStr=boolean  PortDimensions=1  SampleTime=8.33333333333333e-09
  address : Inport  Port=3  OutDataTypeStr=fixdt(0, 11, 0)  PortDimensions=1  SampleTime=8.33333333333333e-09
  edge : Inport  Port=4  OutDataTypeStr=boolean  PortDimensions=1  SampleTime=8.33333333333333e-09
  AND : Logic  IconShape=distinctive  AllPortsSameDT=off  OutDataTypeStr=boolean
  Add : Sum  OutDataTypeStr=fixdt(0, ceil(log2(maxRho*2)), 0)
  Bit Concat : hdlsllib/Logic and Bit Operations/Bit Concat  numInputs=2
      settings: SourceProductName=Simulink
  Bit Slice : hdlsllib/Logic and Bit Operations/Bit Slice  lidx=voteWL-1  ridx=0
  Bitwise AND : simulink/Logic and Bit Operations/Bitwise Operator  logicop=AND  UseBitMask=off  NumInputPorts=2  BitMask=bin2dec('11011001')  BitMaskRealWorld=Stored Integer
  Bitwise NOT : simulink/Logic and Bit Operations/Bitwise Operator  logicop=NOT  UseBitMask=off  BitMask=bin2dec('11011001')  BitMaskRealWorld=Stored Integer
  Bitwise OR : simulink/Logic and Bit Operations/Bitwise Operator  logicop=OR  UseBitMask=off  NumInputPorts=2  BitMask=bin2dec('11011001')  BitMaskRealWorld=Stored Integer
  Block RAM : Subsystem
  Constant : Constant  Value=0  OutDataTypeStr=fixdt(0, 36-voteWL, 0)  SampleTime=-1
  Constant1 : Constant  Value=2^(voteWL)-1  OutDataTypeStr=fixdt(0, 36, 0)  SampleTime=-1
  Delay{,1..2,4..5} (5 alike) : Delay  DelayLength=1
  Multiport Switch : MultiPortSwitch  DataPortOrder=Zero-based contiguous  Inputs=2  zeroidx=on
  Multiport Switch1 : MultiPortSwitch  DataPortOrder=Zero-based contiguous  Inputs=2  zeroidx=on
  Relational Operator : RelationalOperator  Operator===  OutDataTypeStr=boolean  RndMeth=Simplest
  Shift Arithmetic : ArithShift  BitShiftNumberSource=Input port  BitShiftNumber=8  BitShiftDirection=Left  DiagnosticForOORShift=Error
      settings: InputPortMap=u0,p1
  Shift Arithmetic1 : ArithShift  BitShiftNumberSource=Input port  BitShiftNumber=8  BitShiftDirection=Left  DiagnosticForOORShift=Error
      settings: InputPortMap=u0,p1
  Shift Arithmetic2 : ArithShift  BitShiftNumberSource=Input port  BitShiftNumber=8  BitShiftDirection=Right  DiagnosticForOORShift=Error
      settings: InputPortMap=u0,p1
  Signal Specification : SignalSpecification  OutDataTypeStr=fixdt(0, 36, 0)
  Vote : Constant  OutDataTypeStr=fixdt(0,1,0)  SampleTime=-1
  Zero : Constant  Value=0  OutDataTypeStr=fixdt(0,1,0)  SampleTime=-1
  hps : Outport
  wires:
  Block RAM/1(rd_data) -> Signal Specification/1
  Multiport Switch1/1 -> Shift Arithmetic2/1, Bitwise AND/2
  Signal Specification/1 -> Multiport Switch1/2
  Bitwise OR/1 -> Block RAM/1(wr_data), Delay5/1
  Bitwise AND/1 -> Bitwise OR/1
  Shift Arithmetic2/1 -> Bit Slice/1
  Add/1 -> Multiport Switch/3
  Multiport Switch/1 -> Bit Concat/2
  Bit Concat/1 -> Shift Arithmetic/1
  Shift Arithmetic/1 -> Bitwise OR/2
  Delay5/1 -> Multiport Switch1/3
  edge/1 -> Delay1/1
  address/1 -> Block RAM/4(rd_addr), Delay/1, Relational Operator/2
  mode/1 -> Multiport Switch/1
  shift/1 -> Delay4/1
  AND/1 -> Delay2/1
  Bit Slice/1 -> Add/2, hps/1
  Bitwise NOT/1 -> Bitwise AND/1
  Constant/1 -> Bit Concat/1
  Constant1/1 -> Shift Arithmetic1/1
  Delay/1 -> Block RAM/2(wr_addr), Relational Operator/1
  Delay1/1 -> Block RAM/3(wr_en), AND/1
  Delay2/1 -> Multiport Switch1/1
  Delay4/1 -> Shift Arithmetic2/2, Shift Arithmetic/2, Shift Arithmetic1/2
  Relational Operator/1 -> AND/2
  Shift Arithmetic1/1 -> Bitwise NOT/1
  Vote/1 -> Add/1
  Zero/1 -> Multiport Switch/2
